simulink library "lib_exmp"  (R2016a)
settings: Solver=ode45  StartTime=0.0  StopTime=10.0  RelTol=1e-3
values from neighbouring files (symbols this model uses):
  Inertia = eye(3)    [Dynamic_Dependant_control.m]
  q0 = qt/norm(qt)    [Dynamic_Dependant_control.m]
  w0 = rand(3,1)    [Dynamic_Dependant_control.m]
libraries: dspinverses x1, vrlib x1
settings Model: Creator=devantormey  LastModifiedBy=devantormey
settings DataIOCC: LimitDataPoints=on
settings DebuggingCC: AllowSymbolicDim=off

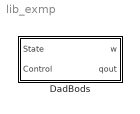
== system lib_exmp ==
  "DadBods " : Subsystem

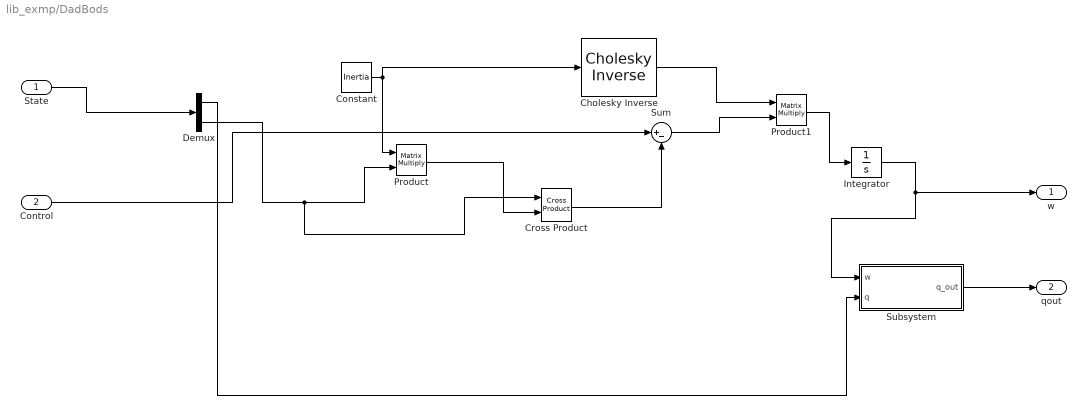
== system lib_exmp/DadBods  ==
  State : Inport
  Control : Inport  Port=2
  Cholesky Inverse : dspinverses/Cholesky Inverse  errmode=Warning
  Constant : Constant  Value=Inertia
  Cross Product : vrlib/Utilities/Cross Product
  Demux : Demux  Outputs=[4 3]
  Integrator : Integrator  InitialCondition=w0
  Product : Product  Multiplication=Matrix(*)
  Product1 : Product  Multiplication=Matrix(*)
  Subsystem : Subsystem
  Sum : Sum  Inputs=|+-
  w : Outport
  qout : Outport  Port=2
  wires:
  State/1 -> Demux/1
  Demux/2 -> Cross Product/1, Product/2
  Constant/1 -> Product/1, Cholesky Inverse/1
  Product/1 -> Cross Product/2
  Control/1 -> Sum/1
  Cross Product/1 -> Sum/2
  Sum/1 -> Product1/2
  Cholesky Inverse/1 -> Product1/1
  Product1/1 -> Integrator/1
  Integrator/1 -> Subsystem/1(w), w/1
  Demux/1 -> Subsystem/2(q)
  Subsystem/1(q_out) -> qout/1

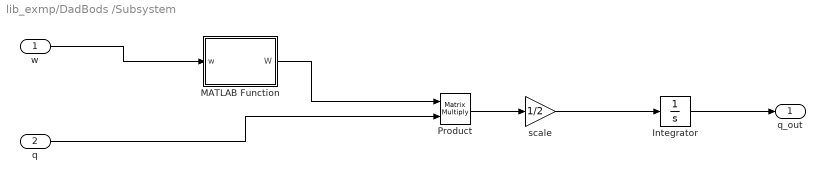
== system lib_exmp/DadBods /Subsystem ==
  w : Inport
  q : Inport  Port=2
  Integrator : Integrator  InitialCondition=q0
  MATLAB Function : MATLAB Function  TreatAsAtomicUnit=on
  Product : Product  Multiplication=Matrix(*)
  scale : Gain  Gain=1/2
  q_out : Outport
  wires:
  w/1 -> MATLAB Function/1(w)
  MATLAB Function/1(W) -> Product/1
  q/1 -> Product/2
  Product/1 -> scale/1
  scale/1 -> Integrator/1
  Integrator/1 -> q_out/1

== matlab function lib_exmp/DadBods /Subsystem/MATLAB Function ==
  data: w input; W output
function W = fcn(w)
%#codegen

W = [0, -w(1),-w(2),-w(3); w(1), 0,w(3), -w(2); w(2), -w(3), 0, w(1); w(3), w(2), -w(1), 0 ];

end
